simulink model "understandingOf_switchBlock"  (R2024b)
settings: Solver=VariableStepAuto  StartTime=0.0  StopTime=10.0  MaxStep=0.01  RelTol=1e-3
settings Model: Creator=admin  LastModifiedBy=admin

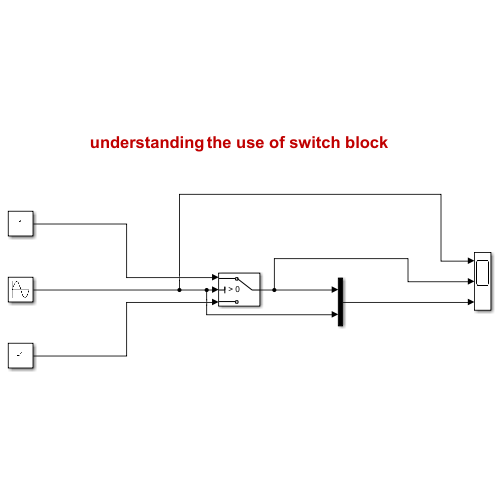
[thumbnail: Simulink's stored preview of the top-level diagram]
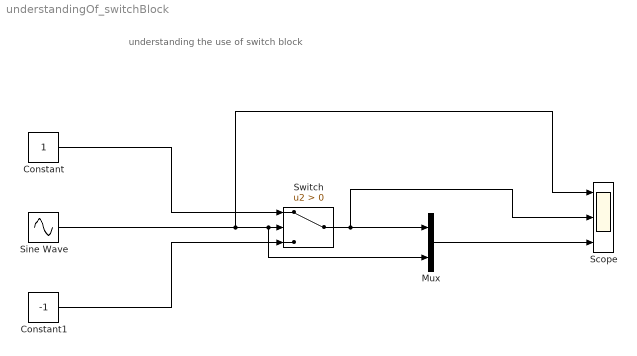
== system understandingOf_switchBlock ==
  note: understanding the use of switch block
  Constant : Constant
  Constant1 : Constant  Value=-1
  Mux : Mux  Inputs=2
  Scope : Scope  NumInputPorts=3
  Sine Wave : Sin  SampleTime=0
  Switch : Switch  Criteria=u2 > Threshold  SaturateOnIntegerOverflow=off  InputSameDT=off
  wires:
  Constant/1 -> Switch/1
  Constant1/1 -> Switch/3
  Switch/1 -> Scope/2, Mux/1
  Mux/1 -> Scope/3
  Sine Wave/1 -> Scope/1, Mux/2, Switch/2
